simulink model "pen_mpcpd"  (R2022b)
settings: Solver=VariableStepAuto  StartTime=0.0  StopTime=20  RelTol=1e-3  AbsTol=1e-3
settings Model: Creator=Abhijit  LastModifiedBy=abhij
settings SolverCC: AutoScaleAbsTol=off  AlgebraicLoopSolver=TrustRegion  MaxZcPerStep=1
settings DebuggingCC: UnconnectedInputMsg=warning  UnconnectedOutputMsg=warning  UnconnectedLineMsg=warning  SymbolicDimsDataTypeCodeGenerationDiagnostic=none  SFMachineParentedDataDiag=warning
settings ModelReferenceCC: EnableRefExpFcnMdlSchedulingChecks=on
settings SFSimCC: CustomCodeUndefinedFunction=UseInterfaceOnly
settings RTWCC: DLArmComputeVersion=19.05
settings SimscapeCC: SimscapeLogType=all  SimscapeLogSimulationStatistics=on  SimscapeLogDataHistory=10000

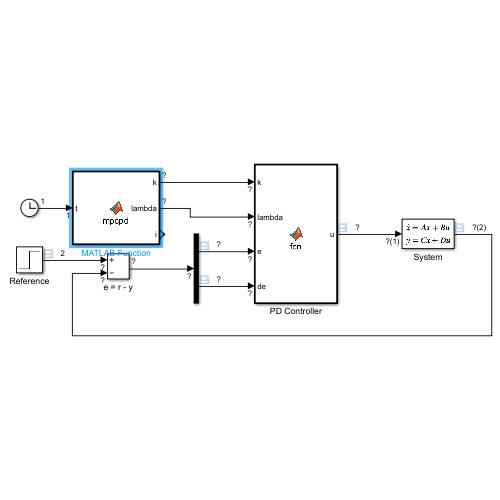
[thumbnail: Simulink's stored preview of the top-level diagram]
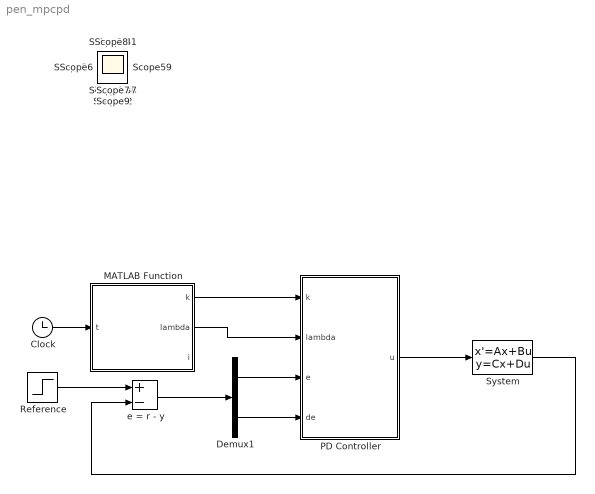
== system pen_mpcpd ==
  Clock : Clock
  Demux1 : Demux  Outputs=2
  MATLAB Function : MATLAB Function  TreatAsAtomicUnit=on
  PD Controller : MATLAB Function  TreatAsAtomicUnit=on
  Reference : Step  Before=[0; 0]  After=[0; pi]  SampleTime=0
  System : StateSpace  A=[0 -1; 1 0]  B=[1; 0]  C=[1 0; 0 1]  D=[0; 0]  InitialCondition=[0; 0]
  e = r - y : Sum  Inputs=+-
  Scope{,1..42} (43 alike) : Scope
  wires:
  System/1 -> e = r - y/2
  Reference/1 -> e = r - y/1
  Demux1/1 -> PD Controller/3(e)
  Demux1/2 -> PD Controller/4(de)
  e = r - y/1 -> Demux1/1
  MATLAB Function/1(k) -> PD Controller/1(k)
  MATLAB Function/2(lambda) -> PD Controller/2(lambda)
  PD Controller/1(u) -> System/1
  Clock/1 -> MATLAB Function/1(t)

== matlab function pen_mpcpd/MATLAB Function ==
  data: t input; k output; lambda output; i output
function [k, lambda, i] = mpcpd(t)
    coder.extrinsic('sim')
    coder.extrinsic('timeseries')

    persistent t_seq u_seq

    %simulation parameters
    model_name = 'pen_mpcpd_offline';

    %horizons
    pred_horizon = 5;
    cont_horizon = 2;
    
    %learning parameters
    u_next_0 = [1; 1];
    du = [0.05; 0.05];
    iterations = 10;
    eta = 0.05;

    %initialise time and control sequences
    if isempty(t_seq)
        t_seq = [0];
        u_seq = [0;0];
    end

    if mod(t, cont_horizon) == 0
        %extend time sequence
        t_seq = [t_seq t];
    
        %copy and extend actual control sequence for gradient descent
        test_seq = u_seq;
        test_seq = [test_seq zeros(2, 1)];
    
        %initialise guess and cost
        u_next = u_next_0;
    
        %perform gradient descent
        for i = 1:iterations   
            %C(k, lambda)
            test_seq(:, end) = u_next;
            C0 = evaluateC(model_name, test_seq, t_seq, t, pred_horizon);
    
            %C(k+dk, lambda)
            test_seq(:, end) = u_next + [du(1); 0];
            Ck = evaluateC(model_name, test_seq, t_seq, t, pred_horizon);
    
            %C(k, lambda+dlambda)
            test_seq(:, end) = u_next + [0; du(2)];
            Clambda = evaluateC(model_name, test_seq, t_seq, t, pred_horizon);
    
            %evaluate gradC
            gradC = [(Ck - C0); (Clambda-C0)]./du;
            
            %step down gradient
            u_next = u_next - eta*gradC;
        end
    
        %extend actual control sequence
        u_seq = [u_seq u_next];
    end

    k = u_seq(1, end);
    lambda = u_seq(2, end);

    function C = evaluateC(mdl_name, u_u_seq, u_t_seq, t_cur, t_extra)
        %construct individual time series for k, lambda
        k_series = timeseries(u_u_seq(1, :), u_t_seq);
        lambda_series = timeseries(u_u_seq(2, :), u_t_seq);
    
        %add time series to base workspace for access by simulink
        assignin('base','k_series', k_series);
        assignin('base','lambda_series', lambda_series);
    
        %simulate
        disp('Sim Started')
        out = sim(mdl_name, t_cur+t_extra);
        disp('Sim Complete')
    
        %get output data and trim to only after current time
        ts = out.tout;
        es = getdatasamples(out.es, 1:length(ts));
        ys = getdatasamples(out.ys, 1:length(ts));
        ts = ts(ts > t_cur);
        es = es(ts > t_cur);
        ys = ys(ts > t_cur);
        
        %calculate cost
        cost = cumtrapz(ts, es.^2 + ys.^2);
        C = cost(end);
    end
end

== matlab function pen_mpcpd/PD Controller ==
  data: k input; lambda input; e input; u output; de input
function u = fcn(k, lambda, e, de)
    u = k*e + lambda*de;
end
